simulink model "sum8"  (R2020b)
settings: Solver=VariableStepAuto  StartTime=0.0  StopTime=10.0  RelTol=1e-3
settings Model: Creator=Shivani  LastModifiedBy=Shivani

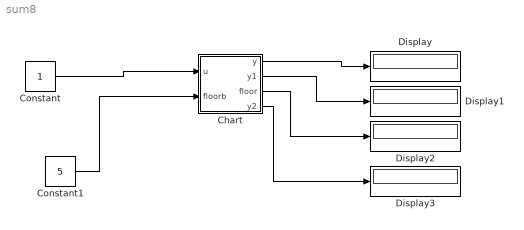
== system sum8 ==
  Chart : Stateflow chart  TreatAsAtomicUnit=on
  Constant : Constant
  Constant1 : Constant  Value=5
  Display{,1..3} (4 alike) : Display
  wires:
  Constant1/1 -> Chart/2(floorb)
  Chart/4(y2) -> Display3/1
  Chart/3(floor) -> Display2/1
  Constant/1 -> Chart/1(u)
  Chart/2(y1) -> Display1/1
  Chart/1(y) -> Display/1

== stateflow chart sum8/Chart ==
  state E_ON
    entry: y = 1;
    state Delay1
      entry:
      floor=floor-1
    state DOWN
      entry:
      floor=floor-1;
    state IDLE
      entry: y1=0;
    state DoorO1
      entry: y2=1;
    state DoorC1
      entry: y2=0;
    state UP
      entry:
      floor=floor+1;
    state Delay
      entry:
      floor=floor+1;
    state DoorO
      entry: y2=1;
    state DoorC
      entry: y2=0;
    (default) -> IDLE
    DOWN -> Delay1 [order 1] : [floorb<floor]
    IDLE -> DOWN [order 2] : [floorb<floor]{y1=1}
    Delay1 -> DOWN [order 1] : [floorb<floor]
    DOWN -> DoorO1 [order 2] : [floorb==floor]
    Delay1 -> DoorO1 [order 2] : [floor==floor]
    IDLE -> UP [order 1] : [floorb>floor]{y1=1}
    DoorO1 -> DoorC1 : after(5,sec)
    Delay -> UP [order 1] : [floorb>floor]
    UP -> Delay [order 2] : [floorb>floor]
    Delay -> DoorO [order 2] : [floor==floorb]
    UP -> DoorO [order 1] : [floorb==floor]
    DoorO -> DoorC : after(500,sec)
  state E_OFF
    entry: y = 0;
  (default) -> E_ON
  E_ON -> E_OFF : [u==0]
  E_OFF -> E_ON : [u==1]
  data: u input; y output [0..1]; floorb input; y1 output [0..1]; floor output [0..5] =0; y2 output
